simulink library "MCHP_Blockset"  (R2014b)
settings: Solver=ode45  SolverMode=SingleTasking  StartTime=0.0  StopTime=10.0  RelTol=1e-3
InitFcn:
  | disp('MCHP_Blockset_Library_InitFunction');
undefined symbols (not defined in the file): A0, A2, AD0, AVdd, B1, B5, B9, C10, C2, CMP2A, CMP3A, CMP4A, EXTREF1, EXTREF2, gcbh, MaxPer, MCHP_ACC_SAMx_Callback, MCHP_ADC_Callback, MCHP_ADC_HighSpeed_SAR_Callback, MCHP_ADC_HighSpeed_SAR_dsPIC_Callback, MCHP_ADC_SAME5x_Callback, MCHP_AFEC_SAM7x_Callback, MCHP_BUS_I2C_MASTER_callback, MCHP_BUS_SPI_callback, MCHP_C_function_Call_callback, MCHP_CN_Callback, MCHP_COMPARATOR1_callback, MCHP_CompilerOptimisation_Callback, MCHP_DACC_SAMx_Callback, MCHP_Digital_Input_Callback, MCHP_Digital_Output_Read_Callback, MCHP_Digital_Output_Write_Callback, MCHP_Fun, MCHP_HighSpeed_AnalogComparator_Callback, MCHP_IC_Callback, MCHP_IdleTask_Callback, MCHP_Interrupt_Callback, MCHP_Master_Callback, MCHP_MCPWM_Callback, MCHP_MCU_LOAD_Callback, MCHP_MCU_OVERLOAD_Callback, MCHP_MSI_Callback, MCHP_OC_HW_Callback, MCHP_OC_SW_Callback, MCHP_OP_AMP_Callback, MCHP_OrderInOut, MCHP_PDEC_Callback, MCHP_PGA_Callback, MCHP_PWM_Callback, MCHP_PWM_HighSpeed_Override_Callback, MCHP_PWM_HS_FEP_Callback, MCHP_PWM_SAM7x_Callback, MCHP_PWM_SAM7x_Override_Callback, MCHP_QDEC_SAMx_Callback, MCHP_QEI_Callback, MCHP_Scheduler_Options_Callback, MCHP_SECONDARY_CORE_Callback, MCHP_Tasks_State_Callback, MCHP_TCC_PWM_Callback, MCHP_TIMER_Config_Callback ... (+18)
libraries: MCHP_Blockset x2
(part 1 of 9)
Description:
  | MPLAB Device Blocks for Simulink.
  | Support for Microchip MCU families:
  |  + dsPIC
  |  + PIC32
  |  + SAMx7
  |  + SAMx5
  |  + SAMx2
settings Model: ModifiedByFormat=Lubin Kerhuel  Creator=Lubin Kerhuel  LastModifiedBy=Lubin Kerhuel

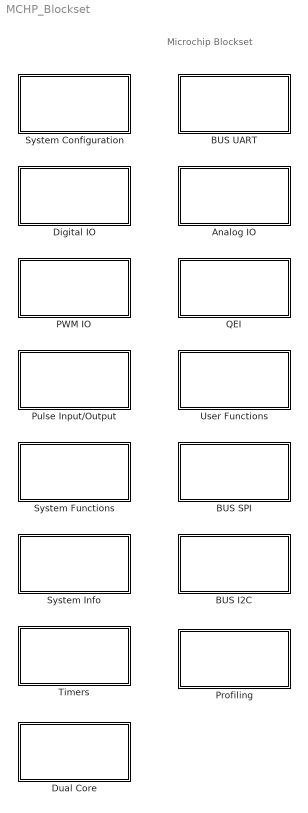
== system MCHP_Blockset ==
  note: Microchip Blockset
  Analog IO : Subsystem
      mask Display:
      | MCHP_DrawLogo;
      | fprintf('Analog\nInput / Output');
  BUS I2C : Subsystem
      mask Display:
      | MCHP_DrawLogo;
      | fprintf('BUS I2C');
  BUS SPI : Subsystem
      mask Display:
      | MCHP_DrawLogo;
      | fprintf('BUS SPI');
  BUS UART : Subsystem
      mask Display:
      | MCHP_DrawLogo;
      | fprintf('BUS UART')
  Digital IO : Subsystem
      mask Display:
      | MCHP_DrawLogo;
      | fprintf('Digital\nInput / Output')
  Dual Core : Subsystem
      mask Display:
      | MCHP_DrawLogo;
      | fprintf('Dual Core')
  PWM IO : Subsystem
      mask Display:
      | MCHP_DrawLogo;
      | fprintf('PWM\nInput / Output');
  Profiling : Subsystem
      mask Display:
      | MCHP_DrawLogo;
      | fprintf('Profiling');
  Pulse Input/Output : Subsystem
      mask Display:
      | MCHP_DrawLogo;
      | fprintf('Pulse \n Input / Output');
  QEI : Subsystem
      mask Display:
      | MCHP_DrawLogo;
      | fprintf('Quadrature Encoder \n Interface');
  System Configuration : Subsystem
      mask Display:
      | MCHP_DrawLogo;
      | fprintf('System\nConfiguration')
  System Functions : Subsystem
      mask Display:
      | MCHP_DrawLogo;
      | disp('System\nFunctions')
  System Info : Subsystem
      mask Display:
      | MCHP_DrawLogo;
      | fprintf('System\nInfo')
  Timers : Subsystem
      mask Display:
      | MCHP_DrawLogo;
      | fprintf('Timers')
  User Functions : Subsystem
      mask Display:
      | MCHP_DrawLogo;
      | disp('User defined\nfunctions')
